simulink model "STATCOM_ssc_Ccode"  (R2024b)
settings: Solver=FixedStepDiscrete  StartTime=0.0  StopTime=2  FixedStep=Ts  RelTol=1e-3  EnableMultiTasking=on
PostLoadFcn:
  | Ts=25e-6; Rsnu=500; Csnu=0.1e-6;
InitFcn:
  | Ts=25e-6; Rsnu=500; Csnu=0.1e-6;
undefined symbols (not defined in the file): DiscIntNeverNeededParam
libraries: ee_lib x19, simetran x14, fl_lib x12, nesl_utility x12, spsSecondOrderFilterLib x3, spsabctodq0Lib x2, simulink x1, spsMeanVariableFrequencyLib x1
(part 1 of 3)
settings Model: Creator=The MathWorks, Inc.  LastModifiedBy=CD8435
settings SolverCC: AlgebraicLoopSolver=TrustRegion
settings DataIOCC: SaveFinalState=on  SaveFormat=StructureWithTime  SaveOutput=off  SaveTime=off  ReturnWorkspaceOutputs=off  SignalLoggingName=sigsOut
settings OptimizationCC: BlockReduction=off  BooleanDataType=off  ExpressionDepthLimit=2147483647  ZeroExternalMemoryAtStartup=off  ZeroInternalMemoryAtStartup=off  InitFltsAndDblsToZero=on  EfficientMapNaN2IntZero=off  LifeSpan=inf
settings DebuggingCC: SaveWithParameterizedLinksMsg=none  UnderspecifiedInitializationDetection=Classic  MergeDetectMultiDrivingBlocksExec=none  CheckExecutionContextPreStartOutputMsg=on  SignalResolutionControl=TryResolveAllWithWarning  MultiTaskDSMMsg=warning  MultiTaskCondExecSysMsg=none  FcnCallInpInsideContextMsg=warning  StateNameClashWarn=warning  SubsystemReferenceDiagnosticForUnitTest=warning  SFUnexpectedBacktrackingDiag=warning  SFNoUnconditionalDefaultTransitionDiag=warning  SFExecutionAtInitializationDiag=none  ArithmeticOperatorsInVariantConditions=warning
settings HardwareCC: ProdBitPerPointer=32  ProdBitPerSizeT=32  ProdBitPerPtrDiffT=32  ProdLargestAtomicFloat=None  ProdIntDivRoundTo=Undefined  ProdEndianess=Unspecified  ProdWordSize=32  ProdHWDeviceType=32-bit Generic  TargetBitPerPointer=64  TargetBitPerSizeT=64  TargetBitPerPtrDiffT=64  TargetLongLongMode=on  TargetIntDivRoundTo=Zero  TargetEndianess=LittleEndian  TargetWordSize=64  TargetHWDeviceType=MATLAB Host  ProdEqTarget=off
settings ModelReferenceCC: EnableRefExpFcnMdlSchedulingChecks=on  PropagateSignalLabelsOutOfModel=off
settings SFSimCC: SimUseLocalCustomCode=off  CustomCodeUndefinedFunction=UseInterfaceOnly
settings RTWCC: RTWUseLocalCustomCode=off  TargetLang=C++  GPUComputeCapability=3.5  DLArmComputeVersion=19.05
settings CodeAppCC: StateflowObjectComments=on
settings GRTTargetCC: TargetFcnLib=ansi_tfl_tmw.mat  TargetLangStandard=C++11 (ISO)  MatFileLogging=off  CodeInterfacePackaging=C++ class
settings ConfigComp: CovMetricSettings=dw  CovSaveCumulativeToWorkspaceVar=on  CovSaveSingleToWorkspaceVar=on  CovExternalEMLEnable=off  CovSFcnEnable=off
settings SimscapeCC: SimscapeNormalizeSystem=off

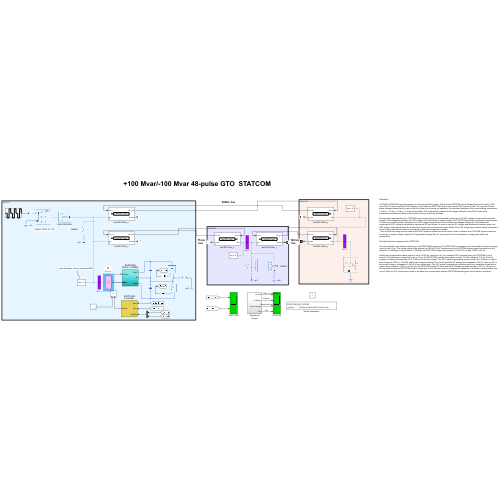
[thumbnail: Simulink's stored preview of the top-level diagram]
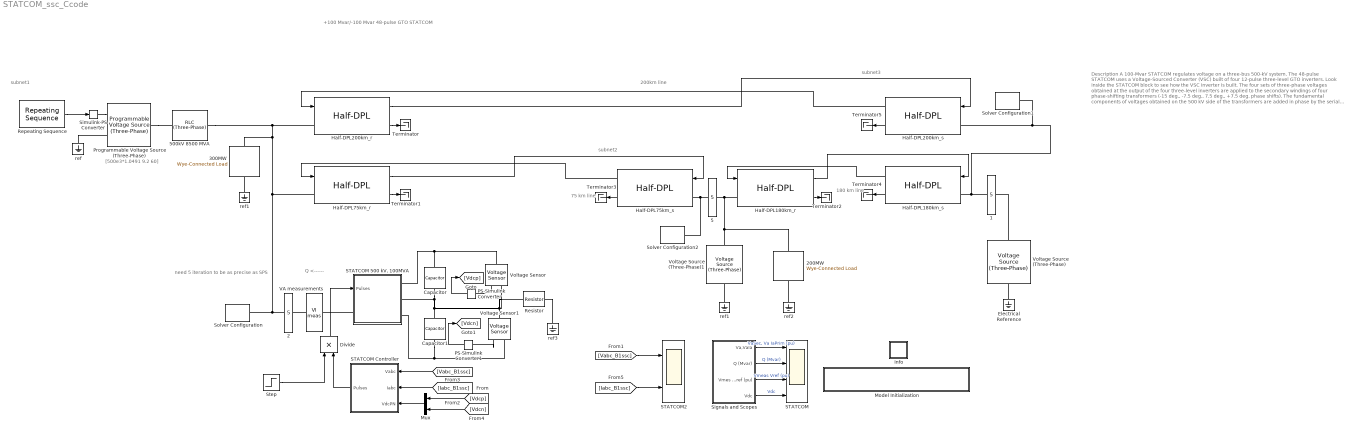
== system STATCOM_ssc_Ccode ==
  note: Description
      |
      |  A 100-Mvar STATCOM regulates voltage on a three-bus 500-kV system. The 48-pulse STATCOM uses a Voltage-Sourced Converter (VSC) built of four 12-pulse three-level GTO inverters. Look inside the STATCOM block to see how the VSC inverter is built. The four sets of three-phase voltages obtained at the output of the four three-level inverters are applied to the secondary windings of four phase-shifting transformers (-15 deg., -7.5 deg., 7.5 deg., +7.5 deg. phase shifts). The fundamental components of voltages obtained on the 500 kV side of the transformers are added in phase by the serial connection of primary windings.
      |
      | During steady-state operation the STATCOM control system keeps the fundamental component of the VSC voltage in phase with the system voltage. If the voltage generated by the VSC is higher (or lower) than the system voltage, the STATCOM generates (or absorbs) reactive power. The amount of reactive power depends on the VSC voltage magnitude and on the transformer leakage reactances. The fundamental component of VSC voltage is controlled by varying the DC bus voltage. In order to vary the DC voltage, and therefore the reactive power, the VSC voltage angle (alpha) which is normally kept close to zero is temporarily phase shifted. This VSC voltage lag or lead produces a temporary flow of active power which results in an increase or decrease of capacitor voltages.
      |   One of the three voltage sources used in the 500 kV system equivalents can be varied in order to observe the STATCOM dynamic response to changes in system voltage. Open the "Programmable Voltage Source" menu and look at the sequence of voltage steps which are programmed.
      |
      | Simulation Dynamic response of the STATCOM
      |
      |  Run the simulation and observe waveforms on the STATCOM scope block. The STATCOM is in voltage control mode and its reference voltage is set to Vref=1.0 pu. The voltage droop of the regulator is 0.03 pu/100 VA.Therefore when the STATCOM operating point changes from fully capacitive (+100 Mvar) to fully inductive (-100 Mvar) the STATCOM voltage varies between 1-0.03=0.97 pu and 1+0.03=1.03 pu.
      |
      | Initially the programmable voltage source is set at 1.0491 pu, resulting in a 1.0 pu voltage at SVC terminals when the STATCOM is out of service. As the reference voltage Vref is set to 1.0 pu, the STATCOM is initially floating (zero current). The DC voltage is 19.3 kV. At t=0.1s, voltage is suddenly decreased by 4.5 % (0.955 pu of nominal voltage). The SVC reacts by generating reactive power (Q=+70 Mvar) in order to keep voltage at 0.979 pu. The 95% settling time is approximately 47 ms. At this point the DC voltage has increased to 20.4 kV. Then, at t=0.2 s the source voltage is increased to1.045 pu of its nominal value. The SVC reacts by changing its operating point from capacitive to inductive in order to keep voltage at 1.021 pu. At this point the STATCOM absorbs 72 Mvar and the DC voltage has been lowered to 18.2 kV. Observe on the first trace showing the STATCOM primary voltage and current that the current is changing from capacitive to inductive in approximately one cycle. Finally, at t=0.3 s the source voltage in set back to its nominal value and the STATCOM operating point comes back to zero Mvar.
  note: 200km line
  note: subnet1
  note: subnet2
  note: subnet3
  note: +100 Mvar/-100 Mvar 48-pulse GTO STATCOM
  note: Q
      | <------
  note: [500e3*1.0491 9.2 60]
  note: need 5 iteration to be as precise as SPS
  note: 75 km
      | line
  note: 180 km
      | line
   ref{,1..3} (4 alike) : fl_lib/Electrical/Electrical Elements/Electrical Reference
  1 : simetran/5  bn=3
      settings: AttributesFormatString=Bus %<bn>
  2 : simetran/5  bn=1
      settings: AttributesFormatString=Bus %<bn>
  200MW : ee_lib/Passive/RLC Assemblies/Wye-Connected Load  port_option=ee.enum.threePhasePort.composite  parameterization=ee.enum.rlc.parameterization.ratedpower  component_structure=ee.enum.rlc.structure.R  component_structure_PQ=ee.enum.rlc.structure.R  R=1 Ohm  L=1e-3 H  C=1e-6 F  VRated=500e3 V  FRated=60 Hz  P=200e6 W  Qpos=1e2 A*V  Qneg=-1e2 A*V  R_parasitic=1e-6 Ohm  G_parasitic=1e-6 1/Ohm  R_parasitic_PQ=1e-6 Ohm  G_parasitic_PQ=1e-6 1/Ohm  Vmag0=24e3 V  Vang0=0 deg  Freq0=60 Hz  IL_specify=off  IL_priority=High  IL=[0, 0, 0] A  IL_nominal_specify=off  IL_nominal_value=1  IL_nominal_unit=A  VC_specify=off  VC_priority=High  VC=[0, 0, 0] V  VC_nominal_specify=off  VC_nominal_value=1  VC_nominal_unit=V
  300MW : ee_lib/Passive/RLC Assemblies/Wye-Connected Load  port_option=ee.enum.threePhasePort.composite  parameterization=ee.enum.rlc.parameterization.ratedpower  component_structure=ee.enum.rlc.structure.R  component_structure_PQ=ee.enum.rlc.structure.R  R=1 Ohm  L=1e-3 H  C=1e-6 F  VRated=500e3 V  FRated=60 Hz  P=300e6 W  Qpos=1e2 A*V  Qneg=-1e2 A*V  R_parasitic=1e-6 Ohm  G_parasitic=1e-6 1/Ohm  R_parasitic_PQ=1e-6 Ohm  G_parasitic_PQ=1e-6 1/Ohm  Vmag0=24e3 V  Vang0=0 deg  Freq0=60 Hz  IL_specify=off  IL_priority=High  IL=[0, 0, 0] A  IL_nominal_specify=off  IL_nominal_value=1  IL_nominal_unit=A  VC_specify=off  VC_priority=High  VC=[0, 0, 0] V  VC_nominal_specify=off  VC_nominal_value=1  VC_nominal_unit=V
  5 : simetran/5  bn=2
      settings: AttributesFormatString=Bus %<bn>
  500kV 8500 MVA : ee_lib/Passive/RLC Assemblies/RLC (Three-Phase)  port_option=ee.enum.threePhasePort.composite  component_structure=ee.enum.rlc.structure.SeriesRL  R=500e3^2/8500e6/10 Ohm  L=500e3^2/8500e6/(2*pi*60) H  C=1e-6 F  R_parasitic=0 Ohm  G_parasitic=0 1/Ohm  IL_specify=off  IL_priority=High  IL=[0, 0, 0] A  IL_nominal_specify=off  IL_nominal_value=1  IL_nominal_unit=A  VC_specify=off  VC_priority=High  VC=[0, 0, 0] V  VC_nominal_specify=off  VC_nominal_value=1  VC_nominal_unit=V
      settings: InternalSimscapePortConfiguration="{\"Bottom\":[],\"Left\":[{\"id\":\"N1\",\"label\":\"~1\",\"type\":\"foundation.electrical.three_phase\"}],\"Right\":[{\"id\":\"N2\",\"label\":\"~2\",\"type\":\"foundation.electrical.three_phase\"}],\"Top\":[]}"
  Capacitor : ee_lib/Passive/Capacitor  cap_option=ee.enum.passive.capacitor.capOption.const  c=3000e-6 F  Cvec=[1e-05, 1e-06] F  Vvec=[0, 10] V  CV_table_symmetry=ee.enum.passive.capacitor.tableSymmetry.yes  f_vec=[1, 10] kHz  DFext_vec=[.8, 1.2]  enable_C_tol=ee.enum.toleranceApplication.none  averaging_period=0 s  C_tol=5  tol_distribution=ee.enum.toleranceDistribution.uniform  nSigma=4  r=0 Ohm  g=0 1/Ohm  enable_operating_limits=ee.enum.enable.no  operating_limit_action=ee.enum.passive.reportOpLim.warn  max_working_voltage_range=[-25, 25] V  power_rating=1 W  maxTemperature=85 degC  thermalEnable=false  thermalMass=1 J/K  fault_action=simscape.enum.assert.action.none  t_fault=1 s  i_specify=off  i_priority=None  i=0 A  i_nominal_specify=off  i_nominal_value=1  i_nominal_unit=A  v_specify=off  v_priority=None  v=10000 V  v_nominal_specify=off  v_nominal_value=1  v_nominal_unit=V  vc_specify=off  vc_priority=High  vc=10000 V  vc_nominal_specify=off  vc_nominal_value=1  vc_nominal_unit=V  T_specify=off  T_priority=None  T=298.15 K  T_nominal_specify=off  T_nominal_value=1  T_nominal_unit=K
  Capacitor1 : ee_lib/Passive/Capacitor  cap_option=ee.enum.passive.capacitor.capOption.const  c=3000e-6 F  Cvec=[1e-05, 1e-06] F  Vvec=[0, 10] V  CV_table_symmetry=ee.enum.passive.capacitor.tableSymmetry.yes  f_vec=[1, 10] kHz  DFext_vec=[.8, 1.2]  enable_C_tol=ee.enum.toleranceApplication.none  averaging_period=0 s  C_tol=5  tol_distribution=ee.enum.toleranceDistribution.uniform  nSigma=4  r=0 Ohm  g=0 1/Ohm  enable_operating_limits=ee.enum.enable.no  operating_limit_action=ee.enum.passive.reportOpLim.warn  max_working_voltage_range=[-25, 25] V  power_rating=1 W  maxTemperature=85 degC  thermalEnable=false  thermalMass=1 J/K  fault_action=simscape.enum.assert.action.none  t_fault=1 s  i_specify=off  i_priority=None  i=0 A  i_nominal_specify=off  i_nominal_value=1  i_nominal_unit=A  v_specify=off  v_priority=None  v=0 V  v_nominal_specify=off  v_nominal_value=1  v_nominal_unit=V  vc_specify=off  vc_priority=High  vc=10000 V  vc_nominal_specify=off  vc_nominal_value=1  vc_nominal_unit=V  T_specify=off  T_priority=None  T=298.15 K  T_nominal_specify=off  T_nominal_value=1  T_nominal_unit=K
  Divide : Product
  Electrical Reference : fl_lib/Electrical/Electrical Elements/Electrical Reference
  Half-DPL180km_r : simetran/Half-DPL  Phases=3  Frequency=60  Resistance=[0.01273*2 0.3864]  Inductance="[0.9337e-3  4.1264e-3]"  Capacitance=[12.74e-9 7.751e-9]  Length=180  Ts=Ts
  Half-DPL180km_s : simetran/Half-DPL  Phases=3  Frequency=60  Resistance=[0.01273*2 0.3864]  Inductance="[0.9337e-3  4.1264e-3]"  Capacitance=[12.74e-9 7.751e-9]  Length=180  Ts=Ts
  Half-DPL200km_r : simetran/Half-DPL  Phases=3  Frequency=60  Resistance=[0.01273*2 0.3864]  Inductance="[0.9337e-3  4.1264e-3]"  Capacitance=[12.74e-9 7.751e-9]  Length=200  Ts=Ts
  Half-DPL200km_s : simetran/Half-DPL  Phases=3  Frequency=60  Resistance=[0.01273*2 0.3864]  Inductance="[0.9337e-3  4.1264e-3]"  Capacitance=[12.74e-9 7.751e-9]  Length=200  Ts=Ts
  Half-DPL75km_r : simetran/Half-DPL  Phases=3  Frequency=60  Resistance=[0.01273*2 0.3864]  Inductance="[0.9337e-3  4.1264e-3]"  Capacitance=[12.74e-9 7.751e-9]  Length=75  Ts=Ts
  Half-DPL75km_s : simetran/Half-DPL  Phases=3  Frequency=60  Resistance=[0.01273*2 0.3864]  Inductance="[0.9337e-3  4.1264e-3]"  Capacitance=[12.74e-9 7.751e-9]  Length=75  Ts=Ts
  Info : Subsystem
      settings: OpenFcn="showExample(\"simscapeelectricalsps/STATCOMExample\")"
      mask Display: disp('?')
  Model Initialization : Subsystem  mask(Model Functions){InitFcnX=Ts=25e-6; Rsnu=500; Csnu=0.1e-6;, prel=off, posl=on, inif=on, strf=off}
      mask prompts: InitFcnX "Initialisation"; prel "Preload Function"; posl "PostLoad Function"; inif "InitFcn"; strf "StartFcn"
      mask init:
      | currentBlock = gcb;
      | root = bdroot(currentBlock);
      | 
      | if ~strcmp(get_param(root,'BlockDiagramType'),'library')
      |     if prel==1
      |         set_param(root, 'PreLoadFcn', InitFcnX);
      |     else
      |         set_param(root, 'PreLoadFcn', '');
      |     end
      |     if inif==1
      |         set_param(root, 'InitFcn', InitFcnX);
      |     else
      |         set_param(root, 'InitFcn', '');
      |     end
      |     if strf==1
      |         set_param(root, 'StartFcn', InitFcnX);
      |     else
      |         set_param(root, 'StartFcn', '');
      |     end
      |     if posl==1
      |         set_param(root, 'PostLoadFcn', InitFcnX);
      |     else
      |         set_param(root, 'PostLoadFcn', '');
      |     end
      | end
      | 
      | pos = get_param(currentBlock, 'Position');
      | width = pos(3) - pos(1); height = pos(4) - pos(2);
      | txt = [ upper(root) '\n' '- InitFcn. . . . . '  get_param(root, 'InitFcn') ];
      settings: CopyFcn=set_param(gcb,'LinkStatus','inactive')
      mask Display: text(5, height*0.5, txt, 'horizontalAlignment', 'left', 'verticalAlignment', 'middle') ;
  Mux : Mux  Inputs=2
  PS-Simulink Converter : nesl_utility/PS-Simulink Converter  PhysicalDomain=network_engine_domain  SubClassName=ps_output  LeftPortType=input  RightPortType=output  PseudoPeriodic=off  Frequencies=[]  VectorFormat=inherit  Unit=inherit  AffineConversion=off
  PS-Simulink Converter1 : nesl_utility/PS-Simulink Converter  PhysicalDomain=network_engine_domain  SubClassName=ps_output  LeftPortType=input  RightPortType=output  PseudoPeriodic=off  Frequencies=[]  VectorFormat=inherit  Unit=inherit  AffineConversion=off
  Programmable Voltage Source (Three-Phase) : ee_lib/Sources/Programmable Voltage Source (Three-Phase)  magnitude_type=ee.enum.timechanging.external  vline_rms=500e3*1.0491 V  magn_ramp=1 V/s  magn_step=1 V  magn_modu_magn=1 V  magn_modu_freq=1 Hz  magn_t1=1 s  magn_t2=2 s  frequency_type=ee.enum.timechanging.constant  freq=60 Hz  freq_ramp=1 Hz/s  freq_step=1 Hz  freq_modu_magn=1 Hz  freq_modu_freq=1 Hz  freq_t1=1 s  freq_t2=2 s  phase_type=ee.enum.timechanging.constant  shift=9.2 deg  phase_ramp=1 deg/s  phase_step=1 deg  phase_modu_magn=1 deg  phase_modu_freq=1 Hz  phase_t1=1 s  phase_t2=2 s  impedance_option=0  SShortCircuit=1e6 A*V  XR=15  R=0.01 Ohm  L=3.97e-4 H  G_parasitic=1e-6 1/Ohm  harmonic_option=0  harmonic_orders=[5, 7, 11, 13]  harmonic_ratios=[.1, .1, .1, .1]  harmonic_shifts=[0, 0, 0, 0] deg  harmonic_sequences=[1, 1, 1, 1]  harmonic_t1=-inf s  harmonic_t2=inf s  I_specify=off  I_priority=None  I=[0, 0, 0] A  I_nominal_specify=off  I_nominal_value=1  I_nominal_unit=A  V_specify=off  V_priority=None  V=[0, 0, 0] V  V_nominal_specify=off  V_nominal_value=1  V_nominal_unit=V
      settings: InternalSimscapePortConfiguration="{\"Bottom\":[],\"Left\":[{\"id\":\"ext_magn\",\"label\":\"M\",\"type\":\"input\"},{\"id\":\"n\",\"label\":\"n\",\"type\":\"foundation.electrical.electrical\"}],\"Right\":[{\"id\":\"N\",\"label\":\"~\",\"type\":\"foundation.electrical.three_phase\"}],\"Top\":[]}"
  Repeating Sequence : simulink/Sources/Repeating Sequence  rep_seq_t="[0   0.1   0.1+Ts   0.2     0.2+Ts  0.3-Ts 0.3 ]"  rep_seq_y="[1    1   0.955    0.955    1.045  1.045    1 ]*500e3*1.0491"
  Resistor : ee_lib/Passive/Resistor  R=1e5 Ohm  enable_R_tol=ee.enum.toleranceApplication.none  R_tol=5  tol_distribution=ee.enum.toleranceDistribution.uniform  nSigma=4  enable_operating_limits=ee.enum.enable.no  operating_limit_action=ee.enum.passive.reportOpLim.warn  power_rating=1 W  max_working_voltage=100 V  noise_mode=ee.enum.sources.noise.Disabled  Tdevice=25 degC  sample_time=1e-3 s  repeatability=ee.enum.ic.repeatability.notRepeatable  user_seed=0  auto_seed=1447930733  fault_action=simscape.enum.assert.action.none  t_fault=1 s  power_derating_T1=70 degC  power_derating_T2=155 degC  operating_temperature_range_vec=[-50, 150] degC  alpha=3.93e-3 1/K  Tmeas=25 degC  thermal_mass=100 J/K  temperature_specify=off  temperature_priority=High  temperature=298.15 K  temperature_nominal_specify=off  temperature_nominal_value=1  temperature_nominal_unit=K
  STATCOM : Scope  NumInputPorts=4
  "STATCOM 500 kV, 100MVA" : Subsystem
  STATCOM Controller : Subsystem  mask(STATCOM Controller){OpMode=Voltage regulation, Vref=1.0, Droop=0.03, Qref1=0, Iqref1=0, ParK_V=[12 3000], ParK_I=[5 40], Ts=Ts}
      mask prompts: OpMode "Operation Mode"; Vref "Reference voltage Vref (pu)"; Droop "Droop (pu/100 MVA):"; Qref1 "Reactive power setpoint Qref (pu)"; Iqref1 "Reactive current setpoint  Iqref (pu):"; ParK_V "Voltage regulator gains: [ Kp  Ki ]"; ParK_I "Iq regulator gains: [ Kp  Ki ]"; Ts "Sample time:"
      mask help:
      | This block implements a controller for a STATCOM using a 48-pulse inverter consisting of  four 3-level bridges and four phase-shifting transformers. The 'Pulses' output is a vectorized signal of the 48 pulses sent to the four 3-level inverters.
      | In Voltage control mode the primary voltage (Vabc) is controlled at Vref within the droop setting. In Var control mode, either the reactive power output or the reactive current is kept constant at Qref (Qref>0 for capacitive mode) or Iqref (Iqref>0 for capacitive mode) .
      mask init:
      | Kp_I=ParK_I(1);
      | Ki_I=ParK_I(2);
      | Kp_V=ParK_V(1);
      | Ki_V=ParK_V(2);
      mask TypeOptions OpMode: Voltage regulation | Var control (Fixed Qref) | Var control (Fixed Iqref)
  STATCOM2 : Scope  NumInputPorts=2
  Signals and Scopes : Subsystem
  Simulink-PS Converter : nesl_utility/Simulink-PS Converter  PhysicalDomain=network_engine_domain  SubClassName=ps_input  LeftPortType=input  RightPortType=output  PseudoPeriodic=off  Frequencies=[]  NoiseDistribution=none  NoiseParameters=[]  Unit=1  AffineConversion=off  FilteringAndDerivatives=provide  SimscapeFilterOrder=1  InputFilterTimeConstant=0.001  UdotUserProvided=0
  Solver Configuration : nesl_utility/Solver Configuration  PhysicalDomain=network_engine_domain  SubClassName=solver  LeftPortType=input  RightPortType=generic  Tones=[]  Harmonics=[]  SimulateNoise=off  Profile=off  UseLocalSampling=off  EnableSwitchedLinearOptims=on  FrequencyDomain=off  UseCCode=off  RelTol=0.001  AbsTol=0.001  MinStep=1e-09  ToWorkspace=off  RevertToSquareIcSolve=off  NumHomotopyIterations=100  PhasorMode=off  PhasorModeNumHarmonics=1  ConsistencySolver=NEWTON_XTOL_AFTER_FTOL  IndexReductionMethod=DerivativeReplacement  DoDC=off  ResidualTolerance=1e-09  ConsistencyTolSource=LOCAL  ConsistencyAbsTol=0.001  ConsistencyRelTol=0.001  ConsistencyTolFactor=0.001  UseLocalSolver=on  LocalSolverChoice=NE_TRAPEZOIDAL_ADVANCER  ResolveIndetEquations=off  FunctionEvalNumThread=1  LocalSolverSampleTime=Ts  DoFixedCost=on  MaxNonlinIter=1  MaxModeIter=2  ComputeImpulses=off  ImpulseIterations=2  LinearAlgebra=auto  LinearAlgebraNumThread=0  EquationFormulation=NE_TIME_EF  DelaysMemoryBudget=1024  AutomaticFiltering=on  FilteringTimeConstant=0.001  PartitionStorageMethod=AS_NEEDED  PartitionMemoryBudget=1024  PartitionMethod=ROBUST  MultibodyUseLocalSolver=off  MultibodyLocalSolverChoice=ODE1  MultibodyLocalSolverSampleTime=0.001
  Solver Configuration1 : nesl_utility/Solver Configuration  PhysicalDomain=network_engine_domain  SubClassName=solver  LeftPortType=input  RightPortType=generic  Tones=[]  Harmonics=[]  SimulateNoise=off  Profile=off  UseLocalSampling=off  EnableSwitchedLinearOptims=on  FrequencyDomain=off  UseCCode=off  RelTol=0.001  AbsTol=0.001  MinStep=1e-09  ToWorkspace=off  RevertToSquareIcSolve=off  NumHomotopyIterations=100  PhasorMode=off  PhasorModeNumHarmonics=1  ConsistencySolver=NEWTON_XTOL_AFTER_FTOL  IndexReductionMethod=DerivativeReplacement  DoDC=off  ResidualTolerance=1e-09  ConsistencyTolSource=GLOBAL  ConsistencyAbsTol=0.001  ConsistencyRelTol=0.001  ConsistencyTolFactor=0.001  UseLocalSolver=on  LocalSolverChoice=NE_BACKWARD_EULER_ADVANCER  ResolveIndetEquations=off  FunctionEvalNumThread=1  LocalSolverSampleTime=Ts  DoFixedCost=on  MaxNonlinIter=1  MaxModeIter=2  ComputeImpulses=off  ImpulseIterations=2  LinearAlgebra=auto  LinearAlgebraNumThread=0  EquationFormulation=NE_TIME_EF  DelaysMemoryBudget=1024  AutomaticFiltering=on  FilteringTimeConstant=0.001  PartitionStorageMethod=AS_NEEDED  PartitionMemoryBudget=1024  PartitionMethod=ROBUST  MultibodyUseLocalSolver=off  MultibodyLocalSolverChoice=ODE1  MultibodyLocalSolverSampleTime=0.001
  Solver Configuration2 : nesl_utility/Solver Configuration  PhysicalDomain=network_engine_domain  SubClassName=solver  LeftPortType=input  RightPortType=generic  Tones=[]  Harmonics=[]  SimulateNoise=off  Profile=off  UseLocalSampling=off  EnableSwitchedLinearOptims=on  FrequencyDomain=off  UseCCode=off  RelTol=0.001  AbsTol=0.001  MinStep=1e-09  ToWorkspace=off  RevertToSquareIcSolve=off  NumHomotopyIterations=100  PhasorMode=off  PhasorModeNumHarmonics=1  ConsistencySolver=NEWTON_XTOL_AFTER_FTOL  IndexReductionMethod=DerivativeReplacement  DoDC=off  ResidualTolerance=1e-09  ConsistencyTolSource=GLOBAL  ConsistencyAbsTol=0.001  ConsistencyRelTol=0.001  ConsistencyTolFactor=0.001  UseLocalSolver=on  LocalSolverChoice=NE_BACKWARD_EULER_ADVANCER  ResolveIndetEquations=off  FunctionEvalNumThread=1  LocalSolverSampleTime=Ts  DoFixedCost=on  MaxNonlinIter=1  MaxModeIter=2  ComputeImpulses=off  ImpulseIterations=2  LinearAlgebra=auto  LinearAlgebraNumThread=0  EquationFormulation=NE_TIME_EF  DelaysMemoryBudget=1024  AutomaticFiltering=on  FilteringTimeConstant=0.001  PartitionStorageMethod=AS_NEEDED  PartitionMemoryBudget=1024  PartitionMethod=ROBUST  MultibodyUseLocalSolver=off  MultibodyLocalSolverChoice=ODE1  MultibodyLocalSolverSampleTime=0.001
  Step : Step  Time=1.5  Before=1  After=0  SampleTime=0
  Terminator{,1..5} (6 alike) : Terminator
  VA measurements : simetran/VI meas  VoltageMeasurement=phase-to-ground  SetLabelV=on  LabelV=Vabc_B1ssc  Vpu=on  VpuLL=off  CurrentMeasurement=yes  SetLabelI=on  LabelI=Iabc_B1ssc  Ipu=on  Pbase=100e6  Vbase=500e3
  Voltage Source (Three-Phase) : ee_lib/Sources/Voltage Source (Three-Phase)  vline_rms=500e3*0.98 V  shift=9.2-40 deg  freq=60 Hz  impedance_option=1  SShortCircuit=9000e6/0.98 A*V  XR=10  R=0.01 Ohm  L=3.97e-4 H  harmonic_option=0  harmonic_orders=[5, 7, 11, 13]  harmonic_ratios=[.1, .1, .1, .1]  G_parasitic=0 1/Ohm  I_specify=off  I_priority=None  I=[0, 0, 0] A  I_nominal_specify=off  I_nominal_value=1  I_nominal_unit=A
  Voltage Source (Three-Phase)1 : ee_lib/Sources/Voltage Source (Three-Phase)  vline_rms=500e3 V  shift=9.2-20 deg  freq=60 Hz  impedance_option=1  SShortCircuit=6500e6 A*V  XR=8  R=0.01 Ohm  L=3.97e-4 H  harmonic_option=0  harmonic_orders=[5, 7, 11, 13]  harmonic_ratios=[.1, .1, .1, .1]  G_parasitic=0 1/Ohm  I_specify=off  I_priority=None  I=[0, 0, 0] A  I_nominal_specify=off  I_nominal_value=1  I_nominal_unit=A
  Voltage Sensor : fl_lib/Electrical/Electrical Sensors/Voltage Sensor
  Voltage Sensor1 : fl_lib/Electrical/Electrical Sensors/Voltage Sensor
  ref1 : fl_lib/Electrical/Electrical Elements/Electrical Reference
  wires:
  Signals and Scopes/1(Va,VaIa) -> STATCOM/1  "VaSec, Va IaPrim (pu)"
  Signals and Scopes/2("Q (Mvar) ") -> STATCOM/2  "Q (Mvar)"
  Signals and Scopes/3(Vmes Vref (pu)) -> STATCOM/3  "Vmeas Vref (pu)"
  Signals and Scopes/4(Vdc) -> STATCOM/4  "Vdc"
  [Vabc_B1ssc] -> STATCOM2/1
  [Iabc_B1ssc] -> STATCOM2/2
  Half-DPL180km_r/1 -> Half-DPL180km_s/1
  Half-DPL180km_s/1 -> Half-DPL180km_r/1
  Half-DPL200km_r/1 -> Half-DPL200km_s/1
  Half-DPL75km_r/1 -> Half-DPL75km_s/1
  Half-DPL200km_s/1 -> Half-DPL200km_r/1
  [Vabc_B1ssc] -> STATCOM Controller/1(Vabc)
  Mux/1 -> STATCOM Controller/3(VdcPN)
  Half-DPL75km_s/1 -> Half-DPL75km_r/1
  PS-Simulink Converter/1 -> [Vdcp]
  Divide/1 -> "STATCOM 500 kV, 100MVA"/1(Pulses)
  PS-Simulink Converter1/1 -> [Vdcn]
  [Vdcn] -> Mux/2
  Repeating Sequence/1 -> Simulink-PS Converter/1
  Step/1 -> Divide/1
  Half-DPL200km_r/2 -> Terminator/1
  [Vdcp] -> Mux/1
  STATCOM Controller/1(Pulses) -> Divide/2
  [Iabc_B1ssc] -> STATCOM Controller/2(Iabc)
  Half-DPL75km_r/2 -> Terminator1/1
  Half-DPL180km_r/2 -> Terminator2/1
  Half-DPL75km_s/2 -> Terminator3/1
  Half-DPL180km_s/2 -> Terminator4/1
  Half-DPL200km_s/2 -> Terminator5/1
  connections:
  Electrical Reference/LConn1 -- Voltage Source (Three-Phase)/LConn1
  Voltage Source (Three-Phase)/RConn1 -- 1/LConn1
  1/RConn1 -- Solver Configuration1/RConn1 -- Half-DPL200km_s/LConn1 -- Half-DPL180km_s/LConn1
  ref1/LConn1 -- Voltage Source (Three-Phase)1/LConn1
  5/LConn1 -- Half-DPL180km_r/LConn1 -- Voltage Source (Three-Phase)1/RConn1 -- 200MW/LConn1
  " ref2"/LConn1 -- 200MW/RConn1
  5/RConn1 -- Solver Configuration2/RConn1 -- Half-DPL75km_s/LConn1
  " ref1"/LConn1 -- 300MW/RConn1
  Capacitor1/RConn1 -- Voltage Sensor1/RConn2 -- "STATCOM 500 kV, 100MVA"/RConn3
  PS-Simulink Converter/LConn1 -- Voltage Sensor/RConn1
  Simulink-PS Converter/RConn1 -- Programmable Voltage Source (Three-Phase)/LConn1
  Resistor/RConn1 -- " ref3"/LConn1
  Programmable Voltage Source (Three-Phase)/RConn1 -- 500kV 8500 MVA/LConn1
  " ref"/LConn1 -- Programmable Voltage Source (Three-Phase)/LConn2
  Capacitor/RConn1 -- Resistor/LConn1 -- Voltage Sensor/RConn2 -- Voltage Sensor1/LConn1 -- Capacitor1/LConn1 -- "STATCOM 500 kV, 100MVA"/RConn2
  "STATCOM 500 kV, 100MVA"/LConn1 -- VA measurements/RConn1
  Voltage Sensor1/RConn1 -- PS-Simulink Converter1/LConn1
  500kV 8500 MVA/RConn1 -- 2/RConn1 -- Solver Configuration/RConn1 -- Half-DPL75km_r/LConn1 -- 300MW/LConn1 -- Half-DPL200km_r/LConn1
  Capacitor/LConn1 -- Voltage Sensor/LConn1 -- "STATCOM 500 kV, 100MVA"/RConn1
  VA measurements/LConn1 -- 2/LConn1

== system STATCOM_ssc_Ccode/Info ==

== system STATCOM_ssc_Ccode/Model Initialization ==

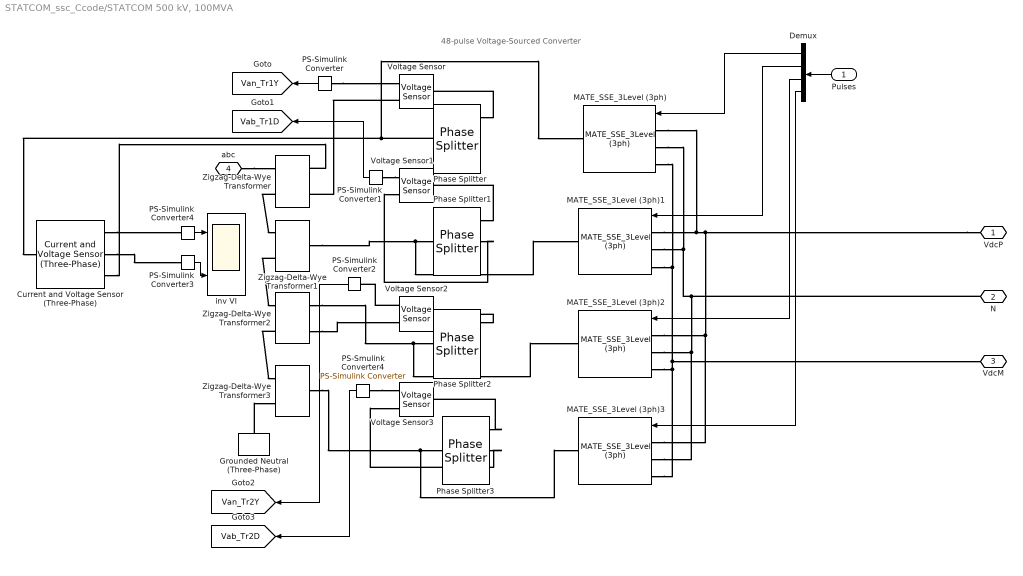
== system STATCOM_ssc_Ccode/STATCOM 500 kV, 100MVA ==
  note: 48-pulse Voltage-Sourced Converter
  Pulses : Inport  PortDimensions=48
  Current and Voltage Sensor (Three-Phase) : ee_lib/Sensors & Transducers/Current and Voltage Sensor (Three-Phase)  vMeasurementType=ee.enum.vmeasurement.ll  outputUnit=ee.enum.unit.si  SRated=100e6 A*V  VRated=24e3 V  I_specify=off  I_priority=None  I=[0, 0, 0] A  I_nominal_specify=off  I_nominal_value=1  I_nominal_unit=A  V_specify=off  V_priority=None  V=[0, 0, 0] V  V_nominal_specify=off  V_nominal_value=1  V_nominal_unit=V
      settings: InternalSimscapePortConfiguration="{\"Bottom\":[],\"Left\":[{\"id\":\"N1\",\"label\":\"~1\",\"type\":\"foundation.electrical.three_phase\"}],\"Right\":[{\"id\":\"V_output\",\"label\":\"V\",\"type\":\"output\"},{\"id\":\"I_output\",\"label\":\"I\",\"type\":\"output\"},{\"id\":\"N2\",\"label\":\"~2\",\"type\":\"foundation.electrical.three_phase\"}],\"Top\":[]}"
  Demux : Demux  Outputs=[12 12 12 12]
      settings: DisplayOption=none
  Grounded Neutral (Three-Phase) : ee_lib/Connectors & References/Grounded Neutral (Three-Phase)
  MATE_SSE_3Level (3ph){,1..3} (4 alike) : simetran/MATE_SSE_3Level (3ph)  SystemSampleTime=-1  VariantActivationTime=update diagram  AllowFlexibleInterface=on  Latency=0  AutoFrameSizeCalculation=off
  PS-Simulink Converter{,1..4} (5 alike) : nesl_utility/PS-Simulink Converter  PhysicalDomain=network_engine_domain  SubClassName=ps_output  LeftPortType=input  RightPortType=output  PseudoPeriodic=off  Frequencies=[]  VectorFormat=inherit  Unit=inherit  AffineConversion=off
  PS-Smulink Converter4 : nesl_utility/PS-Simulink Converter  PhysicalDomain=network_engine_domain  SubClassName=ps_output  LeftPortType=input  RightPortType=output  PseudoPeriodic=off  Frequencies=[]  VectorFormat=inherit  Unit=inherit  AffineConversion=off
  Phase Splitter{,1..3} (4 alike) : ee_lib/Connectors & References/Phase Splitter
  Voltage Sensor{,1..3} (4 alike) : fl_lib/Electrical/Electrical Sensors/Voltage Sensor
  Zigzag-Delta-Wye Transformer : ee_lib/Passive/Transformers/Zigzag-Delta-Wye Transformer  SRated=100e6/4 A*V  FRated=60 Hz  VRated1=500e3/4 V  interconnection_option=ee.enum.zigzaginterconnection.accessibleInterconnects  configuration_option=ee.enum.zigzagconfiguration.Wye  deltaconnection_option=ee.enum.deltaconnection.delta1  VRated2=4160 V  VRated3=15e3 V  phaseShift=7.5 deg  pu_Rw1=0.05/30  pu_Rw2=0.01  pu_Rw3=0.05/30  leakage_reactance_option=ee.enum.transformer_leakage.include  pu_Xl1=0.05  pu_Xl2=0.05  pu_Xl3=0.05  magnetizing_resistance_option=ee.enum.transformer_magnetizingResistance.include  pu_Rm=500  magnetizing_reactance_option=ee.enum.transformer_magnetizingReactance.include  saturation_option=ee.enum.transformer_saturation.exclude  pu_Xm=500  current_data=[0, .1, .25, .5, 1, 2]  magnetic_flux_data=[0, 1, 1.3, 1.45, 1.5, 1.51]  phaseShift_increment=0.1 deg  i1_specify=off  i1_priority=None  i1=[0, 0, 0] A  i1_nominal_specify=off  i1_nominal_value=1  i1_nominal_unit=A  i2_specify=off  i2_priority=None  i2=[0, 0, 0] A  i2_nominal_specify=off  i2_nominal_value=1  i2_nominal_unit=A  i3_specify=off  i3_priority=None  i3=[0, 0, 0] A  i3_nominal_specify=off  i3_nominal_value=1  i3_nominal_unit=A  phi_specify=off  phi_priority=None  phi=[0, 0, 0]  phi_nominal_specify=off  phi_nominal_value=1  phi_nominal_unit=1  power_dissipated_specify=off  power_dissipated_priority=None  power_dissipated=0 W  power_dissipated_nominal_specify=off  power_dissipated_nominal_value=1  power_dissipated_nominal_unit=W
      settings: InternalSimscapePortConfiguration="{\"Bottom\":[],\"Left\":[{\"id\":\"N1\",\"label\":\"~1\",\"type\":\"foundation.electrical.three_phase\"},{\"id\":\"N1n\",\"label\":\"~1i\",\"type\":\"foundation.electrical.three_phase\"}],\"Right\":[{\"id\":\"N3\",\"label\":\"~3\",\"type\":\"foundation.electrical.three_phase\"},{\"id\":\"n3\",\"label\":\"n3\",\"type\":\"foundation.electrical.electrical\"}],\"Top\":[]}"
  Zigzag-Delta-Wye Transformer1 : ee_lib/Passive/Transformers/Zigzag-Delta-Wye Transformer  SRated=100e6/4 A*V  FRated=60 Hz  VRated1=500e3/4 V  interconnection_option=ee.enum.zigzaginterconnection.accessibleInterconnects  configuration_option=ee.enum.zigzagconfiguration.Delta  deltaconnection_option=ee.enum.deltaconnection.delta1  VRated2=15e3 V  VRated3=15e3 V  phaseShift=7.5 deg  pu_Rw1=0.05/30  pu_Rw2=0.05/30  pu_Rw3=0.05/30  leakage_reactance_option=ee.enum.transformer_leakage.include  pu_Xl1=0.05  pu_Xl2=0.05  pu_Xl3=0.05  magnetizing_resistance_option=ee.enum.transformer_magnetizingResistance.include  pu_Rm=500  magnetizing_reactance_option=ee.enum.transformer_magnetizingReactance.include  saturation_option=ee.enum.transformer_saturation.exclude  pu_Xm=500  current_data=[0, .1, .25, .5, 1, 2]  magnetic_flux_data=[0, 1, 1.3, 1.45, 1.5, 1.51]  phaseShift_increment=0.1 deg  i1_specify=off  i1_priority=None  i1=[0, 0, 0] A  i1_nominal_specify=off  i1_nominal_value=1  i1_nominal_unit=A  i2_specify=off  i2_priority=None  i2=[0, 0, 0] A  i2_nominal_specify=off  i2_nominal_value=1  i2_nominal_unit=A  i3_specify=off  i3_priority=None  i3=[0, 0, 0] A  i3_nominal_specify=off  i3_nominal_value=1  i3_nominal_unit=A  phi_specify=off  phi_priority=None  phi=[0, 0, 0]  phi_nominal_specify=off  phi_nominal_value=1  phi_nominal_unit=1  power_dissipated_specify=off  power_dissipated_priority=None  power_dissipated=0 W  power_dissipated_nominal_specify=off  power_dissipated_nominal_value=1  power_dissipated_nominal_unit=W
      settings: InternalSimscapePortConfiguration="{\"Bottom\":[],\"Left\":[{\"id\":\"N1\",\"label\":\"~1\",\"type\":\"foundation.electrical.three_phase\"},{\"id\":\"N1n\",\"label\":\"~1i\",\"type\":\"foundation.electrical.three_phase\"}],\"Right\":[{\"id\":\"N2\",\"label\":\"~2\",\"type\":\"foundation.electrical.three_phase\"}],\"Top\":[]}"
  Zigzag-Delta-Wye Transformer2 : ee_lib/Passive/Transformers/Zigzag-Delta-Wye Transformer  SRated=100e6/4 A*V  FRated=60 Hz  VRated1=500e3/4 V  interconnection_option=ee.enum.zigzaginterconnection.accessibleInterconnects  configuration_option=ee.enum.zigzagconfiguration.Wye  deltaconnection_option=ee.enum.deltaconnection.delta1  VRated2=15e3 V  VRated3=15e3 V  phaseShift=-7.5 deg  pu_Rw1=0.05/30  pu_Rw2=0.01  pu_Rw3=0.05/30  leakage_reactance_option=ee.enum.transformer_leakage.include  pu_Xl1=0.05  pu_Xl2=0.05  pu_Xl3=0.05  magnetizing_resistance_option=ee.enum.transformer_magnetizingResistance.include  pu_Rm=500  magnetizing_reactance_option=ee.enum.transformer_magnetizingReactance.include  saturation_option=ee.enum.transformer_saturation.exclude  pu_Xm=500  current_data=[0, .1, .25, .5, 1, 2]  magnetic_flux_data=[0, 1, 1.3, 1.45, 1.5, 1.51]  phaseShift_increment=0.1 deg  i1_specify=off  i1_priority=None  i1=[0, 0, 0] A  i1_nominal_specify=off  i1_nominal_value=1  i1_nominal_unit=A  i2_specify=off  i2_priority=None  i2=[0, 0, 0] A  i2_nominal_specify=off  i2_nominal_value=1  i2_nominal_unit=A  i3_specify=off  i3_priority=None  i3=[0, 0, 0] A  i3_nominal_specify=off  i3_nominal_value=1  i3_nominal_unit=A  phi_specify=off  phi_priority=None  phi=[0, 0, 0]  phi_nominal_specify=off  phi_nominal_value=1  phi_nominal_unit=1  power_dissipated_specify=off  power_dissipated_priority=None  power_dissipated=0 W  power_dissipated_nominal_specify=off  power_dissipated_nominal_value=1  power_dissipated_nominal_unit=W
      settings: InternalSimscapePortConfiguration="{\"Bottom\":[],\"Left\":[{\"id\":\"N1\",\"label\":\"~1\",\"type\":\"foundation.electrical.three_phase\"},{\"id\":\"N1n\",\"label\":\"~1i\",\"type\":\"foundation.electrical.three_phase\"}],\"Right\":[{\"id\":\"N3\",\"label\":\"~3\",\"type\":\"foundation.electrical.three_phase\"},{\"id\":\"n3\",\"label\":\"n3\",\"type\":\"foundation.electrical.electrical\"}],\"Top\":[]}"
  Zigzag-Delta-Wye Transformer3 : ee_lib/Passive/Transformers/Zigzag-Delta-Wye Transformer  SRated=100e6/4 A*V  FRated=60 Hz  VRated1=500e3/4 V  interconnection_option=ee.enum.zigzaginterconnection.accessibleInterconnects  configuration_option=ee.enum.zigzagconfiguration.Delta  deltaconnection_option=ee.enum.deltaconnection.delta1  VRated2=15e3 V  VRated3=15e3 V  phaseShift=-7.5 deg  pu_Rw1=0.05/30  pu_Rw2=0.05/30  pu_Rw3=0.05/30  leakage_reactance_option=ee.enum.transformer_leakage.include  pu_Xl1=0.05  pu_Xl2=0.05  pu_Xl3=0.05  magnetizing_resistance_option=ee.enum.transformer_magnetizingResistance.include  pu_Rm=500  magnetizing_reactance_option=ee.enum.transformer_magnetizingReactance.include  saturation_option=ee.enum.transformer_saturation.exclude  pu_Xm=500  current_data=[0, .1, .25, .5, 1, 2]  magnetic_flux_data=[0, 1, 1.3, 1.45, 1.5, 1.51]  phaseShift_increment=0.1 deg  i1_specify=off  i1_priority=None  i1=[0, 0, 0] A  i1_nominal_specify=off  i1_nominal_value=1  i1_nominal_unit=A  i2_specify=off  i2_priority=None  i2=[0, 0, 0] A  i2_nominal_specify=off  i2_nominal_value=1  i2_nominal_unit=A  i3_specify=off  i3_priority=None  i3=[0, 0, 0] A  i3_nominal_specify=off  i3_nominal_value=1  i3_nominal_unit=A  phi_specify=off  phi_priority=None  phi=[0, 0, 0]  phi_nominal_specify=off  phi_nominal_value=1  phi_nominal_unit=1  power_dissipated_specify=off  power_dissipated_priority=None  power_dissipated=0 W  power_dissipated_nominal_specify=off  power_dissipated_nominal_value=1  power_dissipated_nominal_unit=W
      settings: InternalSimscapePortConfiguration="{\"Bottom\":[],\"Left\":[{\"id\":\"N1\",\"label\":\"~1\",\"type\":\"foundation.electrical.three_phase\"},{\"id\":\"N1n\",\"label\":\"~1i\",\"type\":\"foundation.electrical.three_phase\"}],\"Right\":[{\"id\":\"N2\",\"label\":\"~2\",\"type\":\"foundation.electrical.three_phase\"}],\"Top\":[]}"
  inv VI : Scope  NumInputPorts=2
  VdcP : PMIOPort  Side=Right
  N : PMIOPort  Port=2  Side=Right
  VdcM : PMIOPort  Port=3  Side=Right
  abc : PMIOPort  Port=4  Side=Left
  tag scope: Vab_Tr1D=global, Vab_Tr2D=global, Van_Tr1Y=global, Van_Tr2Y=global
  wires:
  Pulses/1 -> Demux/1
  Demux/1 -> MATE_SSE_3Level (3ph)/1
  Demux/2 -> MATE_SSE_3Level (3ph)1/1
  Demux/3 -> MATE_SSE_3Level (3ph)2/1
  Demux/4 -> MATE_SSE_3Level (3ph)3/1
  PS-Simulink Converter/1 -> [Van_Tr1Y]
  PS-Simulink Converter1/1 -> [Vab_Tr1D]
  PS-Simulink Converter2/1 -> [Van_Tr2Y]
  PS-Smulink Converter4/1 -> [Vab_Tr2D]
  PS-Simulink Converter3/1 -> inv VI/2
  PS-Simulink Converter4/1 -> inv VI/1
  connections:
  Grounded Neutral (Three-Phase)/LConn1 -- Zigzag-Delta-Wye Transformer3/LConn2
  Zigzag-Delta-Wye Transformer2/LConn2 -- Zigzag-Delta-Wye Transformer3/LConn1
  Zigzag-Delta-Wye Transformer1/LConn2 -- Zigzag-Delta-Wye Transformer2/LConn1
  Zigzag-Delta-Wye Transformer/LConn2 -- Zigzag-Delta-Wye Transformer1/LConn1
  abc/RConn1 -- Zigzag-Delta-Wye Transformer/LConn1
  Phase Splitter/RConn1 -- Voltage Sensor/LConn1
  Zigzag-Delta-Wye Transformer1/RConn1 -- MATE_SSE_3Level (3ph)1/RConn1 -- Phase Splitter1/LConn1
  Phase Splitter1/RConn2 -- Voltage Sensor1/RConn2
  Phase Splitter1/RConn1 -- Voltage Sensor1/LConn1
  Phase Splitter2/RConn1 -- Voltage Sensor2/LConn1
  Zigzag-Delta-Wye Transformer2/RConn1 -- MATE_SSE_3Level (3ph)2/RConn1 -- Phase Splitter2/LConn1
  Phase Splitter3/RConn2 -- Voltage Sensor3/RConn2
  Zigzag-Delta-Wye Transformer3/RConn1 -- MATE_SSE_3Level (3ph)3/RConn1 -- Phase Splitter3/LConn1
  Phase Splitter3/RConn1 -- Voltage Sensor3/LConn1
  VdcP/RConn1 -- MATE_SSE_3Level (3ph)1/LConn1 -- MATE_SSE_3Level (3ph)/LConn1 -- MATE_SSE_3Level (3ph)3/LConn1 -- MATE_SSE_3Level (3ph)2/LConn1
  MATE_SSE_3Level (3ph)1/LConn2 -- MATE_SSE_3Level (3ph)/LConn2 -- N/RConn1 -- MATE_SSE_3Level (3ph)3/LConn2 -- MATE_SSE_3Level (3ph)2/LConn2
  MATE_SSE_3Level (3ph)3/LConn3 -- MATE_SSE_3Level (3ph)2/LConn3 -- VdcM/RConn1 -- MATE_SSE_3Level (3ph)1/LConn3 -- MATE_SSE_3Level (3ph)/LConn3
  Voltage Sensor/RConn2 -- Zigzag-Delta-Wye Transformer/RConn2
  PS-Simulink Converter/LConn1 -- Voltage Sensor/RConn1
  PS-Simulink Converter1/LConn1 -- Voltage Sensor1/RConn1
  Zigzag-Delta-Wye Transformer2/RConn2 -- Voltage Sensor2/RConn2
  Voltage Sensor2/RConn1 -- PS-Simulink Converter2/LConn1
  PS-Smulink Converter4/LConn1 -- Voltage Sensor3/RConn1
  Phase Splitter/LConn1 -- MATE_SSE_3Level (3ph)/RConn1 -- Current and Voltage Sensor (Three-Phase)/LConn1
  Current and Voltage Sensor (Three-Phase)/RConn3 -- Zigzag-Delta-Wye Transformer/RConn1
  Current and Voltage Sensor (Three-Phase)/RConn2 -- PS-Simulink Converter3/LConn1
  Current and Voltage Sensor (Three-Phase)/RConn1 -- PS-Simulink Converter4/LConn1

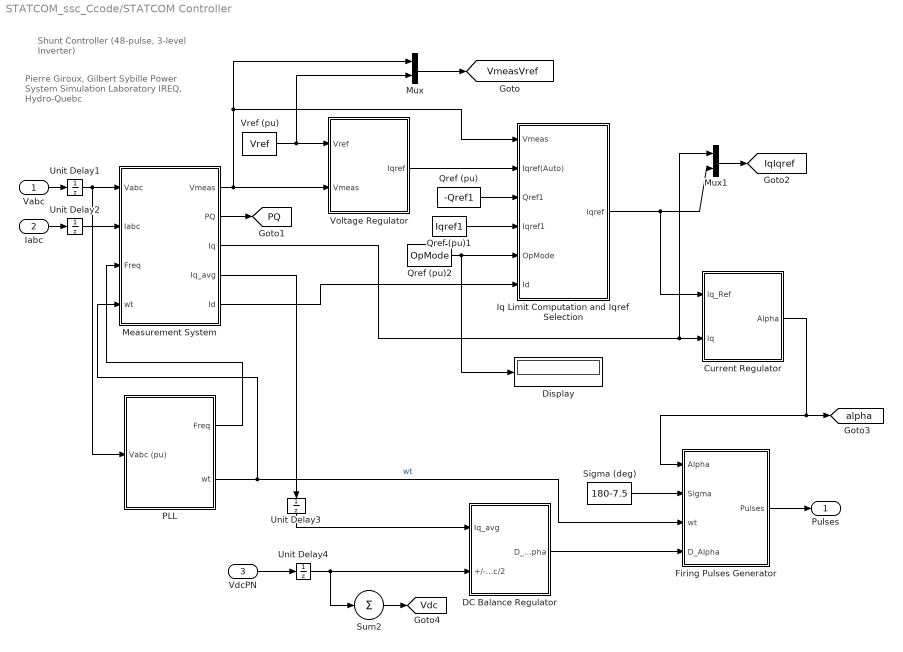
== system STATCOM_ssc_Ccode/STATCOM Controller ==
  note: Shunt Controller
      | (48-pulse, 3-level Inverter)
  note: Pierre Giroux, Gilbert Sybille
      | Power System Simulation Laboratory
      | IREQ, Hydro-Quebc
  Vabc : Inport  PortDimensions=3
  Iabc : Inport  Port=2  PortDimensions=3
  VdcPN : Inport  Port=3  PortDimensions=2
  Current Regulator : Subsystem  mask(Discrete PI Controller){Kp=Kp_I, Ki=Ki_I, Par_Limits=[80 -80], Init=0, Ts=Ts}
      mask prompts: Kp "Proportional gain (Kp):"; Ki "Integral gain (Ki):"; Par_Limits "Output limits: [ Upper   Lower ]"; Init "Output initial value:"; Ts "Sample time:"
      mask help: This block implements a discrete PI controller.
      mask init:
      | UpperLimit=Par_Limits(1);
      | LowerLimit=Par_Limits(2);
  DC Balance Regulator : Subsystem
  Display : Display
  Firing Pulses Generator : Subsystem
  Iq Limit Computation and Iqref Selection : Subsystem
  Measurement System : Subsystem
  Mux : Mux  Inputs=2
  Mux1 : Mux  Inputs=2
  PLL : Subsystem  mask(Discrete 3-phase PLL){Nstep=1, Par_Init=[0 60], ParK=[60 1400], Ts=Ts}
      mask prompts: Nstep "PLL timing correction (in number of time step)"; Par_Init "Initial inputs:[ Phase(degrees)   Frequency(Hz) ]"; ParK "Regulator gains [ Kp  Ki ]"; Ts "Sample time:"
      mask help:
      | This Phase Locked Loop (PLL) system can be used  to synchronize on a set of variable frequency, three-phase sinusoidal signals.
      |
      | Input 1: Vector containing the normalized
      |              three-phase signals [Va Vb Vc]
      | Output 1:  Measured frequency (Hz) = w/(2pi)
      | Output 2:  Ramp w.t   varying between  0 and 2*pi,
      | synchronized on zero crossings of the fundamental (positive-sequence) of phase A.
      | Output 3: Vector [sin(wt) cos(wt)]
      mask init:
      | Kp=ParK(1);
      | Ki=ParK(2);
      | Phase_Init=Par_Init(1);
      | Finit=Par_Init(2);
  Qref (pu) : Constant  Value=-Qref1
  Qref (pu)1 : Constant  Value=Iqref1
  Qref (pu)2 : Constant  Value=OpMode
  Sigma (deg) : Constant  Value=180-7.5
  Sum2 : Sum  Inputs=1  InputSameDT=on  SaturateOnIntegerOverflow=on  OutDataTypeStr=Inherit: Same as first input
  Unit Delay{1..4} (4 alike) : UnitDelay  SampleTime=Ts  HasFrameUpgradeWarning=on
  Voltage Regulator : Subsystem  mask(Discrete PI Controller){Droop=Droop, Kp=Kp_V, Ki=Ki_V, Par_Limits=[1 -1], Init=0, Ts=Ts}
      mask prompts: Droop "Droop (pu/100MVA):"; Kp "Proportional gain (Kp):"; Ki "Integral gain (Ki):"; Par_Limits "Output limits: [ Upper   Lower ]"; Init "Output initial value:"; Ts "Sample time:"
      mask help: This block implements a discrete PI controller.
      mask init:
      | UpperLimit=Par_Limits(1);
      | LowerLimit=Par_Limits(2);
  Vref (pu) : Constant  Value=Vref
  Pulses : Outport  VectorParamsAs1DForOutWhenUnconnected=off
  tag scope: IqIqref=global, PQ=global, Vdc=global, VmeasVref=global, alpha=global
  wires:
  Current Regulator/1(Alpha) -> [alpha], Firing Pulses Generator/1(Alpha)
  Sigma (deg)/1 -> Firing Pulses Generator/2(Sigma)
  Mux1/1 -> [IqIqref]
  Iq Limit Computation and Iqref Selection/1(Iqref) -> Mux1/2, Current Regulator/1(Iq_Ref)
  Vref (pu)/1 -> Mux/2, Voltage Regulator/1(Vref)
  Measurement System/5(Id) -> Iq Limit Computation and Iqref Selection/6(Id)
  Measurement System/3(Iq) -> Mux1/1, Current Regulator/2(Iq)
  Qref (pu)1/1 -> Iq Limit Computation and Iqref Selection/4(Iqref1)
  Qref (pu)/1 -> Iq Limit Computation and Iqref Selection/3(Qref1)
  Measurement System/1(Vmeas) -> Voltage Regulator/2(Vmeas), Iq Limit Computation and Iqref Selection/1(Vmeas), Mux/1
  Measurement System/2(PQ) -> [PQ]
  Voltage Regulator/1(Iqref) -> Iq Limit Computation and Iqref Selection/2(Iqref(Auto))
  Qref (pu)2/1 -> Iq Limit Computation and Iqref Selection/5(OpMode), Display/1
  PLL/1(Freq) -> Measurement System/3(Freq)
  PLL/2(wt) -> Firing Pulses Generator/3(wt), Measurement System/4(wt)  "wt"
  Vabc/1 -> Unit Delay1/1
  Measurement System/4(Iq_avg) -> Unit Delay3/1
  Unit Delay3/1 -> DC Balance Regulator/1(Iq_avg)
  Mux/1 -> [VmeasVref]
  VdcPN/1 -> Unit Delay4/1
  Firing Pulses Generator/1(Pulses) -> Pulses/1
  Iabc/1 -> Unit Delay2/1
  Sum2/1 -> [Vdc]
  Unit Delay1/1 -> PLL/1(Vabc (pu)), Measurement System/1(Vabc)
  Unit Delay2/1 -> Measurement System/2(Iabc)
  Unit Delay4/1 -> DC Balance Regulator/2(+/-Vdc/2), Sum2/1
  DC Balance Regulator/1(D_Alpha) -> Firing Pulses Generator/4(D_Alpha)

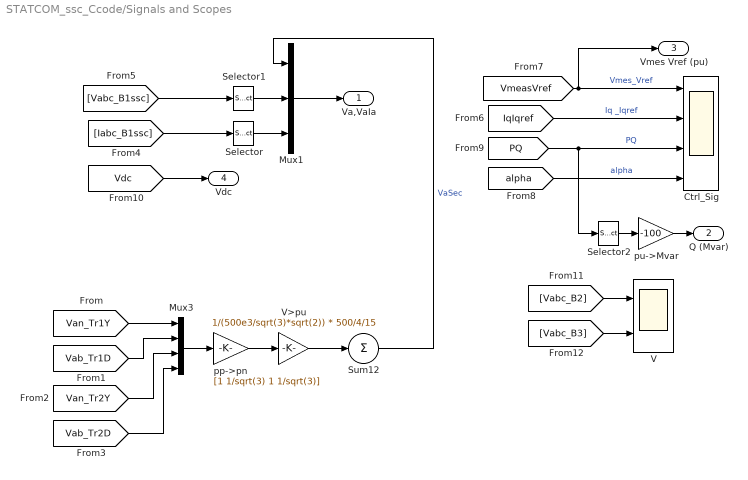
== system STATCOM_ssc_Ccode/Signals and Scopes ==
  Ctrl_Sig : Scope  NumInputPorts=4
  Mux1 : Mux  Inputs=3
  Mux3 : Mux
  Selector : Selector  InputPortWidth=3  IndexOptions=Index vector (dialog)  Indices=1  OutputSizes=1
  Selector1 : Selector  InputPortWidth=3  IndexOptions=Index vector (dialog)  Indices=1  OutputSizes=1
  Selector2 : Selector  InputPortWidth=2  IndexOptions=Index vector (dialog)  Indices=2  OutputSizes=1
  Sum12 : Sum  Inputs=1  InputSameDT=on  SaturateOnIntegerOverflow=on  OutDataTypeStr=Inherit: Same as first input
  V : Scope  NumInputPorts=2
  "V>pu " : Gain  Gain=1/(500e3/sqrt(3)*sqrt(2)) * 500/4/15  SaturateOnIntegerOverflow=on  OutDataTypeStr=Inherit: Same as input  ParamDataTypeStr=Inherit: Same as input
  pp->pn : Gain  Gain=[1 1/sqrt(3) 1 1/sqrt(3)]  SaturateOnIntegerOverflow=on  OutDataTypeStr=Inherit: Same as input  ParamDataTypeStr=Inherit: Same as input
  pu->Mvar : Gain  Gain=-100  SaturateOnIntegerOverflow=on  OutDataTypeStr=Inherit: Same as input  ParamDataTypeStr=Inherit: Same as input
  Va,VaIa : Outport  VectorParamsAs1DForOutWhenUnconnected=off
  "Q (Mvar) " : Outport  Port=2  VectorParamsAs1DForOutWhenUnconnected=off
  Vmes Vref (pu) : Outport  Port=3  VectorParamsAs1DForOutWhenUnconnected=off
  Vdc : Outport  Port=4  VectorParamsAs1DForOutWhenUnconnected=off
  wires:
  "V>pu "/1 -> Sum12/1
  pp->pn/1 -> "V>pu "/1
  Mux3/1 -> pp->pn/1
  [Van_Tr1Y] -> Mux3/1
  [Vab_Tr1D] -> Mux3/2
  [Van_Tr2Y] -> Mux3/3
  [Vab_Tr2D] -> Mux3/4
  Mux1/1 -> Va,VaIa/1
  [VmeasVref] -> Vmes Vref (pu)/1, Ctrl_Sig/1  "Vmes_Vref"
  Selector1/1 -> Mux1/2
  Selector/1 -> Mux1/3
  Sum12/1 -> Mux1/1  "VaSec"
  [IqIqref] -> Ctrl_Sig/2  "Iq _Iqref"
  [PQ] -> Ctrl_Sig/3, Selector2/1  "PQ"
  [alpha] -> Ctrl_Sig/4  "alpha"
  [Vabc_B1ssc] -> Selector1/1
  [Iabc_B1ssc] -> Selector/1
  [Vdc] -> Vdc/1
  [Vabc_B2] -> V/1
  [Vabc_B3] -> V/2
  Selector2/1 -> pu->Mvar/1
  pu->Mvar/1 -> "Q (Mvar) "/1

== system STATCOM_ssc_Ccode/STATCOM Controller/Current Regulator ==
  Iq_Ref : Inport
  Iq : Inport  Port=2
  Discrete-Time Integrator : DiscreteIntegrator  InitialCondition=Init  SampleTime=Ts  LimitOutput=on  UpperSaturationLimit=UpperLimit*10  LowerSaturationLimit=LowerLimit*10  ICPrevOutput=DiscIntNeverNeededParam  ICPrevScaledInput=DiscIntNeverNeededParam
  Kp4 : Gain  Gain=Kp  SaturateOnIntegerOverflow=on  OutDataTypeStr=Inherit: Same as input  ParamDataTypeStr=Inherit: Same as input
  Kp5 : Gain  Gain=Ki  SaturateOnIntegerOverflow=on  OutDataTypeStr=Inherit: Same as input  ParamDataTypeStr=Inherit: Same as input
  Saturation2 : Saturate  UpperLimit=UpperLimit  LowerLimit=LowerLimit
  Sum : Sum  Inputs=-+|  InputSameDT=on  SaturateOnIntegerOverflow=on  OutDataTypeStr=Inherit: Same as first input
  Sum6 : Sum  InputSameDT=on  SaturateOnIntegerOverflow=on  OutDataTypeStr=Inherit: Same as first input
  Alpha : Outport  InitialOutput=0  VectorParamsAs1DForOutWhenUnconnected=off
  wires:
  Iq_Ref/1 -> Sum/1
  Sum6/1 -> Saturation2/1
  Kp5/1 -> Discrete-Time Integrator/1
  Kp4/1 -> Sum6/1
  Discrete-Time Integrator/1 -> Sum6/2
  Saturation2/1 -> Alpha/1
  Iq/1 -> Sum/2
  Sum/1 -> Kp5/1, Kp4/1  "Err"

== system STATCOM_ssc_Ccode/STATCOM Controller/DC Balance Regulator ==
  Iq_avg : Inport  PortDimensions=1
  +/-Vdc/2 : Inport  Port=2  PortDimensions=2
  " Mean value" : Subsystem  mask(Discrete Mean value){Freq=60, Vinit=0, Ts=Ts}
      mask prompts: Freq "Fundamental frequency (Hz):"; Vinit "Initial input (DC component):"; Ts "Sample time:"
      mask help:
      | This block computes the mean value of the input signal over a running window of one cycle of the specified fundamental frequency.
      | For the first cycle of simulation, the output is held constant to the value specified by the parameter "Initial input".
      mask init:
      | SamplesPerCycle=1/Freq/Ts;
      | RoundSamplesPerCycle=round(SamplesPerCycle);
      | Delay=RoundSamplesPerCycle*Ts - Ts/2;
      | Correction=SamplesPerCycle/RoundSamplesPerCycle - 1;
  Abs : Abs
  D_Alpha(Manual) : Constant  Value=0
  D_Alpha1 : Constant  Value=0
  D_Alpha2 : Constant  Value=0
  D_Alpha5 : Constant  Value=0.1
  Demux : Demux  Outputs=2
      settings: DisplayOption=none
  Gain : Gain  Gain=0  SaturateOnIntegerOverflow=on  OutDataTypeStr=Inherit: Same as input  ParamDataTypeStr=Inherit: Same as input
  Gain1 : Gain  Gain=-1  SaturateOnIntegerOverflow=on  OutDataTypeStr=Inherit: Same as input  ParamDataTypeStr=Inherit: Same as input
  Mode : Constant
  Multiport Switch : MultiPortSwitch
  PI Regulator : Subsystem  mask(Discrete PI Controller){Kp=0.001, Ki=0.01, Par_Limits=[2 -2], Init=0, Ts=Ts}
      mask prompts: Kp "Proportional gain (Kp):"; Ki "Integral gain (Ki):"; Par_Limits "Output limits: [ Upper   Lower ]"; Init "Output initial value:"; Ts "Sample time:"
      mask help: This block implements a discrete PI controller.
      mask init:
      | UpperLimit=Par_Limits(1);
      | LowerLimit=Par_Limits(2);
      mask Display: disp('PI');
  Relational Operator : RelationalOperator  Operator=<=
  Relational Operator1 : RelationalOperator  Operator=<
  Sum2 : Sum  Inputs=-+  InputSameDT=on  SaturateOnIntegerOverflow=on  OutDataTypeStr=Inherit: Same as first input
  Switch : Switch  Threshold=0.5
  Switch1 : Switch  Threshold=0.5
  D_Alpha : Outport  VectorParamsAs1DForOutWhenUnconnected=off
  wires:
  Relational Operator1/1 -> PI Regulator/2(Reset), Switch1/2
  Multiport Switch/1 -> D_Alpha/1
  D_Alpha(Manual)/1 -> Multiport Switch/3  "Man"
  PI Regulator/1(Out) -> Gain1/1, Switch/1
  Mode/1 -> Multiport Switch/1
  D_Alpha2/1 -> Multiport Switch/4  "Off"
  Switch/1 -> Multiport Switch/2  "Auto"
  Relational Operator/1 -> Switch/2
  Gain1/1 -> Switch/3
  D_Alpha5/1 -> Relational Operator1/2
  Abs/1 -> Relational Operator1/1
  D_Alpha1/1 -> Relational Operator/2
  " Mean value"/1(Mean) -> Switch1/3, Gain/1
  Gain/1 -> Switch1/1
  Switch1/1 -> PI Regulator/1(Error)
  Sum2/1 -> " Mean value"/1(In)
  Iq_avg/1 -> Abs/1, Relational Operator/1
  +/-Vdc/2/1 -> Demux/1
  Demux/1 -> Sum2/1
  Demux/2 -> Sum2/2
